simulink model "massdamper"  (R2023b)
settings: Solver=VariableStepAuto  StartTime=0.0  StopTime=200  RelTol=1e-3
model workspace (MAT data in the model file):
  PnFrequencyOffset_21 = [30000 100000 1000000 3000000 10000000]
  uniqueString_21 = '90_5792'
values from neighbouring files (symbols this model uses):
  A = [0 1;-K/M -fv/M]    [massdamperml.m]
  B = [0;1/M]    [massdamperml.m]
  C = [1 0]    [massdamperml.m]
  D = 0    [massdamperml.m]
  F = 100    [massdamperml.m]
  fv = 1    [massdamperml.m]
  K = 1    [massdamperml.m]
  M = 2    [massdamperml.m]
  Q = 2.3    [massdamperml.m]
  R = 1    [massdamperml.m]
  Ts = 1    [massdamperml.m]
undefined symbols (not defined in the file or in its folder): Continuous, Time
libraries: simulink x2, ctrlSharedLib x1
settings Model: Creator=bjkgu  LastModifiedBy=bjkgu

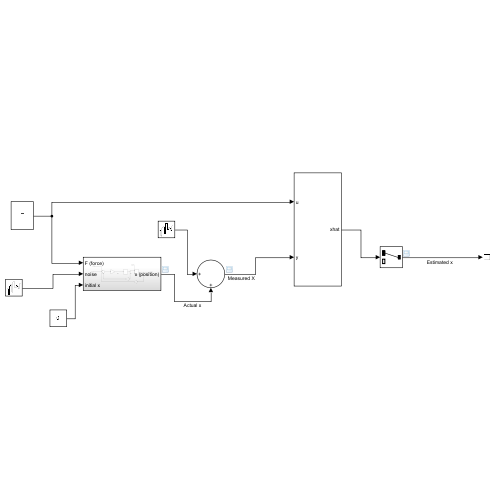
[thumbnail: Simulink's stored preview of the top-level diagram]
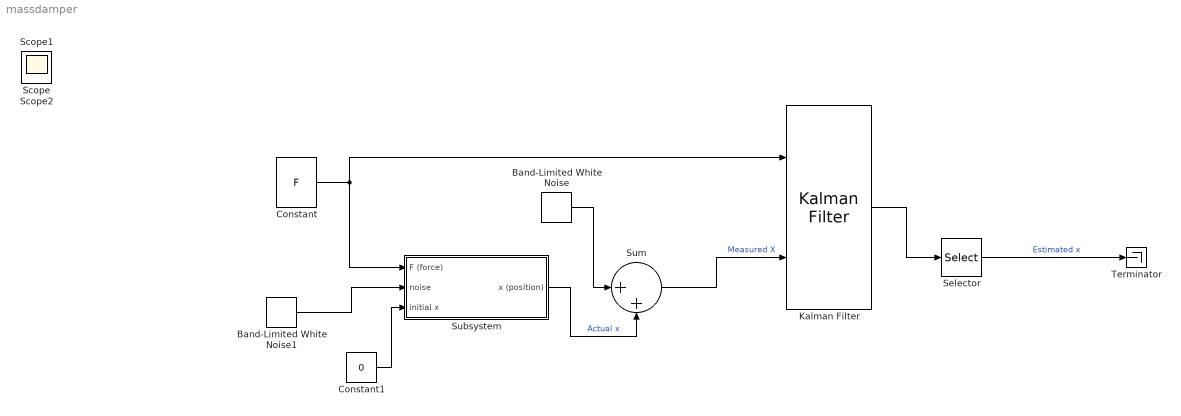
== system massdamper ==
  Band-Limited White Noise : simulink/Sources/Band-Limited White Noise  Cov=R*Ts  Ts=Ts  seed=[23341]
  Band-Limited White Noise1 : simulink/Sources/Band-Limited White Noise  Cov=Q*Ts  Ts=Ts  seed=[23341]
  Constant : Constant  Value=F
  Constant1 : Constant  Value=0
  Kalman Filter : ctrlSharedLib/Kalman Filter  TimeDomain=Continuous-Time  UseCurrentEstimator=on  ModelSource=Individual A, B, C, D matrices  ModelSourceVariable=ss(0.95,1,1,0,1)  A=A  B=B  C=C  D=D  NumberOfStates=1  NumberOfInputs=1  NumberOfOutputs=1  InitialEstimateSource=Dialog  X0=[5 0]  P0=10  UseK=off  UseGH=off  NumberOfProcessNoiseInputs=1  G=1  TimeInvariantG=on  H=0  TimeInvariantH=on  Q=diag([0 Q])  TimeInvariantQ=on  R=R  TimeInvariantR=on  N=0  TimeInvariantN=on  AddInputPort=on  AddEnablePort=off  OutputEstimatedY=off  OutputP=off  Ts=-1
  Selector : Selector  InputPortWidth=2  IndexOptions=Index vector (dialog)  Indices=1  OutputSizes=1
  Subsystem : Subsystem
  Sum : Sum  Inputs=|++
  Terminator : Terminator
  Scope : Scope
  Scope1 : Scope
  Scope2 : Scope
  wires:
  Constant/1 -> Subsystem/1(F (force)), Kalman Filter/1
  Subsystem/1(x (position)) -> Sum/2  "Actual x"
  Band-Limited White Noise/1 -> Sum/1
  Sum/1 -> Kalman Filter/2  "Measured X"
  Kalman Filter/1 -> Selector/1
  Selector/1 -> Terminator/1  "Estimated x"
  Band-Limited White Noise1/1 -> Subsystem/2(noise)
  Constant1/1 -> Subsystem/3(initial x)

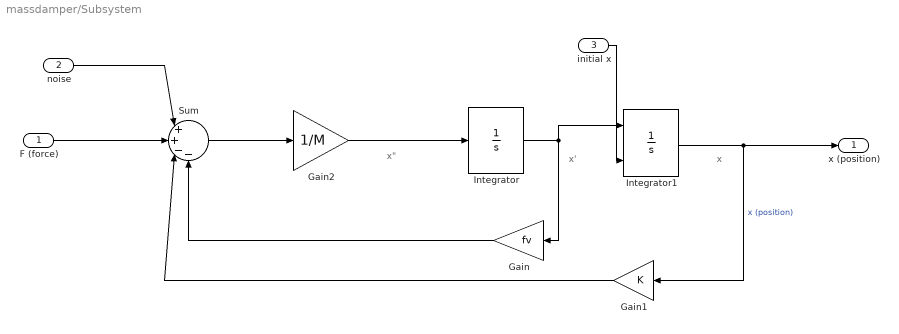
== system massdamper/Subsystem ==
  note: x"
  note: x'
  note: x
  F (force) : Inport
  noise : Inport  Port=2
  initial x : Inport  Port=3
  Gain : Gain  Gain=fv
  Gain1 : Gain  Gain=K
  Gain2 : Gain  Gain=1/M
  Integrator : Integrator
  Integrator1 : Integrator  InitialConditionSource=external
  Sum : Sum  Inputs=|++--
  x (position) : Outport
  wires:
  Sum/1 -> Gain2/1
  Integrator/1 -> Gain/1, Integrator1/1
  Integrator1/1 -> x (position)/1, Gain1/1  "x (position)"
  Gain2/1 -> Integrator/1
  Gain1/1 -> Sum/3
  Gain/1 -> Sum/4
  F (force)/1 -> Sum/2
  noise/1 -> Sum/1
  initial x/1 -> Integrator1/2
